simulink model "OriginalSystem"  (R2016b)
settings: Solver=FixedStepDiscrete  StartTime=0.0  StopTime=100.0  FixedStep=0.05  RelTol=1e-3
undefined symbols (not defined in the file): DiscIntNeverNeededParam
libraries: simulink x1
settings Model: Creator=ASUS  LastModifiedBy=ASUS

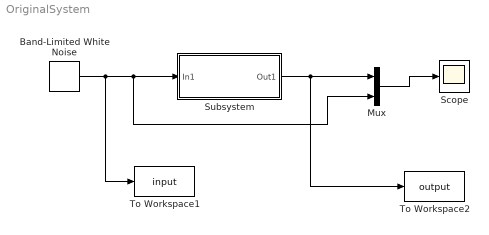
== system OriginalSystem ==
  Band-Limited White Noise : simulink/Sources/Band-Limited White Noise  Cov=[0.1]  Ts=0.05  seed=[23341]
  Mux : Mux  Inputs=2
  Scope : Scope
  Subsystem : Subsystem
  To Workspace1 : ToWorkspace  VariableName=input  SampleTime=-1
  To Workspace2 : ToWorkspace  VariableName=output  SampleTime=-1
  wires:
  Band-Limited White Noise/1 -> To Workspace1/1, Mux/2, Subsystem/1(In1)
  Subsystem/1(Out1) -> To Workspace2/1, Mux/1
  Mux/1 -> Scope/1

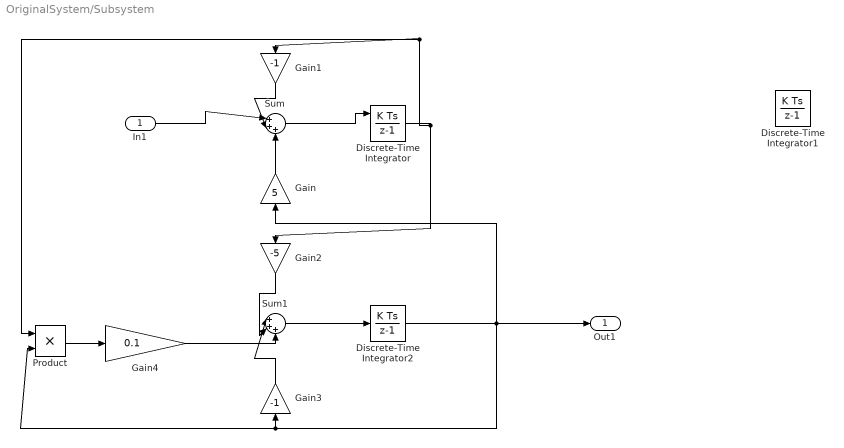
== system OriginalSystem/Subsystem ==
  In1 : Inport
  Discrete-Time Integrator : DiscreteIntegrator  InitialConditionSource=external  InitialConditionSetting=State (most efficient)  SampleTime=-1  ICPrevOutput=DiscIntNeverNeededParam  ICPrevScaledInput=DiscIntNeverNeededParam
  Discrete-Time Integrator1 : DiscreteIntegrator  InitialConditionSetting=State (most efficient)  SampleTime=-1  ICPrevOutput=DiscIntNeverNeededParam  ICPrevScaledInput=DiscIntNeverNeededParam
  Discrete-Time Integrator2 : DiscreteIntegrator  InitialConditionSetting=State (most efficient)  SampleTime=-1  ICPrevOutput=DiscIntNeverNeededParam  ICPrevScaledInput=DiscIntNeverNeededParam
  Gain : Gain  Gain=5
  Gain1 : Gain  Gain=-1
  Gain2 : Gain  Gain=-5
  Gain3 : Gain  Gain=-1
  Gain4 : Gain  Gain=0.1
  Product : Product
  Sum : Sum  Inputs=|+++
  Sum1 : Sum  Inputs=|+++
  Out1 : Outport
  wires:
  In1/1 -> Sum/1
  Gain1/1 -> Sum/2
  Gain/1 -> Sum/3
  Sum/1 -> Discrete-Time Integrator/1
  Gain3/1 -> Sum1/1
  Gain2/1 -> Sum1/2
  Sum1/1 -> Discrete-Time Integrator2/1
  Discrete-Time Integrator2/1 -> Product/2, Gain3/1, Gain/1, Out1/1
  Discrete-Time Integrator/1 -> Product/1, Gain1/1, Gain2/1
  Gain4/1 -> Sum1/3
  Product/1 -> Gain4/1
